simulink model "sampleModel1960"  (R2023a)
settings: Solver=VariableStepAuto  StartTime=0.0  StopTime=10.0  RelTol=1e-3
libraries: hdlsllib x4, simulink x2
settings Model: Creator=user1  LastModifiedBy=user1

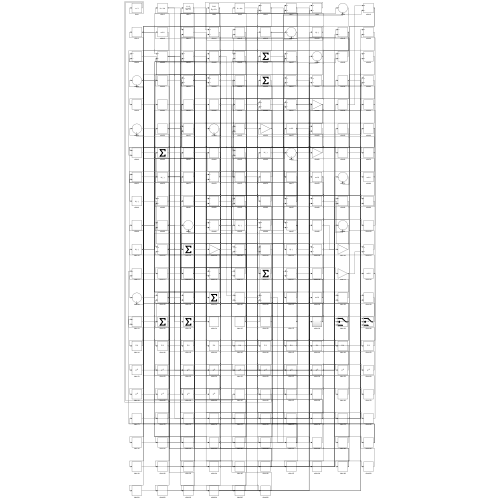
[thumbnail: Simulink's stored preview of the top-level diagram]
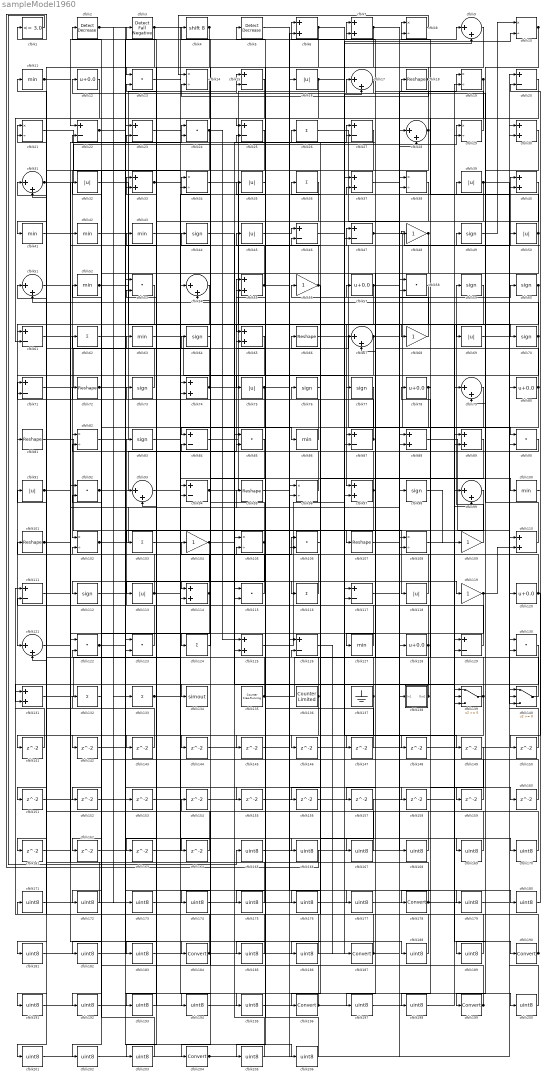
== system sampleModel1960 ==
  cfblk1 : hdlsllib/Logic and Bit Operations/Compare To Constant  relop=<=  const=3.0  OutDataTypeStr=boolean
  cfblk{8,10,14,19,21,29,34,38,82,96,102,105,108} (13 alike) : Product  Inputs=*/  RndMeth=Zero  SaturateOnIntegerOverflow=on
  cfblk{11,41..43,52,63,86,100,127} (9 alike) : MinMax
  cfblk{18,66,72,81,95,101,107} (7 alike) : Reshape
  cfblk{26,36,62,103,116,124,132..133} (8 alike) : Sum  Inputs=+
  cfblk{48,56,68,104,109,119} (6 alike) : Gain
  cfblk{13,24,53,58,85,90,92,106,115,122..123,130} (12 alike) : DotProduct  OutDataTypeStr=Inherit: Inherit via internal rule
  cfblk{6..7,30,33,37,40,55,65,74,88..89,97,110,114,125,131} (16 alike) : Sum
  cfblk{15,20,22..23,25,27,46..47,61,71,84,87,94,111,117,126,129} (17 alike) : Sum  Inputs=+-
  cfblk{44,49,59..60,64,70,73,76..77,83,98,112} (12 alike) : Signum
  cfblk{16,32,35,39,45,50,69,75,91,113,118} (11 alike) : Abs  SaturateOnIntegerOverflow=off
  cfblk{12,57,78,80,120,128} (6 alike) : Bias  Bias=0.0  SaturateOnIntegerOverflow=off
  cfblk{9,17,28,31,51,54,67,79,93,99,121} (11 alike) : Sum  Inputs=|++
  cfblk134 : ToWorkspace  VariableName=simout  SaveFormat=Timeseries  SampleTime=-1
  cfblk135 : hdlsllib/Sources/Counter Free-Running  NumBits=16  tsamp=-1
  cfblk136 : hdlsllib/Sources/Counter Limited  uplimit=7  tsamp=-1
  cfblk137 : Ground
  cfblk138 : Subsystem
      settings: LibrarySourceBlock=|
      | hdlsllib/Ports &
      | Subsystems/Subsystem
  cfblk139 : Switch  SaturateOnIntegerOverflow=off  InputSameDT=off
  cfblk140 : Switch  SaturateOnIntegerOverflow=off  InputSameDT=off
  cfblk{141..164} (24 alike) : Delay  SampleTime=1
  cfblk{165..177,179..183,185..186,188..189,191..195,197..198,200..203,205..206} (35 alike) : DataTypeConversion  OutDataTypeStr=uint8  SaturateOnIntegerOverflow=off  RndMeth=Floor
  cfblk{178,184,187,190,196,199,204} (7 alike) : DataTypeConversion  SaturateOnIntegerOverflow=off  RndMeth=Floor
  cfblk2 : simulink/Logic and Bit Operations/Detect Decrease  vinit=0.0  OutDataTypeStr=boolean
      settings: LibrarySourceBlock=|
      | hdlsllib/Logic and Bit
      | Operations/Detect
      | Decrease
  cfblk3 : hdlsllib/Logic and Bit Operations/Detect Fall Negative  vinit=0  OutDataTypeStr=boolean
  cfblk4 : ArithShift  BitShiftNumber=8
  cfblk5 : simulink/Logic and Bit Operations/Detect Decrease  vinit=0.0  OutDataTypeStr=boolean
      settings: LibrarySourceBlock=|
      | hdlsllib/Logic and Bit
      | Operations/Detect
      | Decrease
  wires:
  cfblk116/1 -> cfblk104/1
  cfblk74/1 -> cfblk17/1, cfblk31/1
  cfblk82/1 -> cfblk15/1
  cfblk98/1 -> cfblk109/1
  cfblk124/1 -> cfblk4/1
  cfblk17/1 -> cfblk15/2
  cfblk123/1 -> cfblk83/1
  cfblk54/1 -> cfblk121/1
  cfblk8/1 -> cfblk14/1
  cfblk47/1 -> cfblk90/1, cfblk19/1
  cfblk68/1 -> cfblk56/1
  cfblk65/1 -> cfblk81/1
  cfblk100/1 -> cfblk48/1
  cfblk66/1 -> cfblk90/2
  cfblk75/1 -> cfblk96/2, cfblk115/2
  cfblk24/1 -> cfblk102/1, cfblk125/1
  cfblk81/1 -> cfblk118/1
  cfblk32/1 -> cfblk97/1
  cfblk34/1 -> cfblk68/1
  cfblk29/1 -> cfblk6/1
  cfblk31/1 -> cfblk29/1, cfblk124/1
  cfblk49/1 -> cfblk10/1
  cfblk136/1 -> cfblk55/2, cfblk191/1
  cfblk87/1 -> cfblk71/1, cfblk46/2
  cfblk30/1 -> cfblk199/1
  cfblk85/1 -> cfblk204/1
  cfblk94/1 -> cfblk10/2, cfblk27/1
  cfblk109/1 -> cfblk59/1
  cfblk92/1 -> cfblk55/1, cfblk133/1
  cfblk61/1 -> cfblk82/1
  cfblk131/1 -> cfblk74/1
  cfblk9/1 -> cfblk25/1
  cfblk78/1 -> cfblk125/2, cfblk148/1
  cfblk76/1 -> cfblk26/1
  cfblk36/1 -> cfblk134/1
  cfblk97/1 -> cfblk23/2, cfblk156/1, cfblk157/1
  cfblk20/1 -> cfblk178/1
  cfblk127/1 -> cfblk93/1
  cfblk120/1 -> cfblk3/1, cfblk150/1
  cfblk22/1 -> cfblk8/2, cfblk153/1, cfblk195/1
  cfblk55/1 -> cfblk45/1, cfblk27/2
  cfblk50/1 -> cfblk8/1, cfblk127/1
  cfblk42/1 -> cfblk129/1
  cfblk28/1 -> cfblk93/2, cfblk18/1
  cfblk64/1 -> cfblk114/1
  cfblk56/1 -> cfblk25/2, cfblk146/1
  cfblk62/1 -> cfblk123/1
  cfblk52/1 -> cfblk120/1, cfblk7/2
  cfblk69/1 -> cfblk110/1
  cfblk86/1 -> cfblk34/1
  cfblk93/1 -> cfblk100/1
  cfblk95/1 -> cfblk47/1
  cfblk140/1 -> cfblk21/1
  cfblk128/1 -> cfblk131/2, cfblk67/2, cfblk101/1
  cfblk96/1 -> cfblk2/1
  cfblk107/1 -> cfblk60/1
  cfblk118/1 -> cfblk76/1
  cfblk114/1 -> cfblk52/1, cfblk182/1
  cfblk103/1 -> cfblk107/1
  cfblk104/1 -> cfblk112/1, cfblk39/1
  cfblk7/1 -> cfblk160/1, cfblk161/1
  cfblk73/1 -> cfblk11/1
  cfblk23/1 -> cfblk34/2
  cfblk88/1 -> cfblk140/3
  cfblk16/1 -> cfblk65/1, cfblk69/1, cfblk9/2
  cfblk26/1 -> cfblk88/1
  cfblk13/1 -> cfblk114/2
  cfblk110/1 -> cfblk12/1
  cfblk119/1 -> cfblk139/2, cfblk110/2
  cfblk84/1 -> cfblk40/1
  cfblk4/1 -> cfblk41/1, cfblk103/1
  cfblk6/1 -> cfblk67/1, cfblk164/1
  cfblk63/1 -> cfblk87/1
  cfblk14/1 -> cfblk113/1
  cfblk122/1 -> cfblk32/1, cfblk158/1
  cfblk3/1 -> cfblk70/1, cfblk151/1
  cfblk108/1 -> cfblk190/1
  cfblk2/1 -> cfblk170/1, cfblk173/1
  cfblk113/1 -> cfblk82/2, cfblk200/1
  cfblk101/1 -> cfblk42/1, cfblk24/2
  cfblk21/1 -> cfblk54/1
  cfblk112/1 -> cfblk119/1
  cfblk121/1 -> cfblk95/1
  cfblk138/1(Out1) -> cfblk122/2, cfblk7/1
  cfblk57/1 -> cfblk159/1, cfblk201/1
  cfblk89/1 -> cfblk196/1
  cfblk44/1 -> cfblk139/3
  cfblk71/1 -> cfblk40/2
  cfblk33/1 -> cfblk97/2, cfblk86/1
  cfblk139/1 -> cfblk66/1, cfblk78/1, cfblk147/1, cfblk185/1
  cfblk67/1 -> cfblk38/2, cfblk77/1
  cfblk111/1 -> cfblk184/1
  cfblk129/1 -> cfblk57/1
  cfblk51/1 -> cfblk129/2
  cfblk125/1 -> cfblk17/2
  cfblk60/1 -> cfblk121/2, cfblk194/1
  cfblk45/1 -> cfblk46/1
  cfblk70/1 -> cfblk75/1, cfblk51/2
  cfblk80/1 -> cfblk84/1, cfblk22/2
  cfblk137/1 -> cfblk51/1, cfblk92/2, cfblk174/1
  cfblk102/1 -> cfblk28/1, cfblk116/1, cfblk162/1
  cfblk72/1 -> cfblk64/1, cfblk106/2, cfblk177/1
  cfblk25/1 -> cfblk61/1
  cfblk39/1 -> cfblk80/1, cfblk54/2
  cfblk10/1 -> cfblk79/2, cfblk189/1
  cfblk41/1 -> cfblk123/2
  cfblk133/1 -> cfblk37/2, cfblk106/1
  cfblk48/1 -> cfblk142/1, cfblk203/1
  cfblk135/1 -> cfblk33/1, cfblk28/2
  cfblk12/1 -> cfblk61/2
  cfblk19/1 -> cfblk94/2, cfblk144/1
  cfblk90/1 -> cfblk84/2
  cfblk18/1 -> cfblk14/2, cfblk13/1
  cfblk91/1 -> cfblk24/1, cfblk49/1
  cfblk115/1 -> cfblk71/2
  cfblk126/1 -> cfblk187/1
  cfblk11/1 -> cfblk22/1, cfblk9/1
  cfblk105/1 -> cfblk44/1, cfblk183/1
  cfblk15/1 -> cfblk141/1
  cfblk141/1 -> cfblk131/1
  cfblk40/1 -> cfblk143/1
  cfblk143/1 -> cfblk21/2
  cfblk144/1 -> cfblk6/2
  cfblk35/1 -> cfblk145/1
  cfblk146/1 -> cfblk79/1
  cfblk147/1 -> cfblk65/2
  cfblk148/1 -> cfblk140/1
  cfblk46/1 -> cfblk149/1
  cfblk150/1 -> cfblk140/2
  cfblk151/1 -> cfblk47/2
  cfblk27/1 -> cfblk152/1
  cfblk152/1 -> cfblk96/1
  cfblk153/1 -> cfblk94/1
  cfblk154/1 -> cfblk139/1
  cfblk43/1 -> cfblk155/1
  cfblk155/1 -> cfblk29/2
  cfblk156/1 -> cfblk38/1
  cfblk158/1 -> cfblk19/2
  cfblk159/1 -> cfblk102/2
  cfblk160/1 -> cfblk105/1
  cfblk77/1 -> cfblk163/1
  cfblk163/1 -> cfblk74/2
  cfblk164/1 -> cfblk31/2
  cfblk1/1 -> cfblk165/1
  cfblk165/1 -> cfblk128/1
  cfblk162/1 -> cfblk166/1
  cfblk166/1 -> cfblk1/1
  cfblk5/1 -> cfblk167/1
  cfblk167/1 -> cfblk35/1
  cfblk37/1 -> cfblk168/1
  cfblk168/1 -> cfblk5/1
  cfblk117/1 -> cfblk169/1
  cfblk169/1 -> cfblk92/1
  cfblk170/1 -> cfblk117/1
  cfblk171/1 -> cfblk117/2
  cfblk130/1 -> cfblk172/1
  cfblk172/1 -> cfblk122/1
  cfblk173/1 -> cfblk130/1
  cfblk174/1 -> cfblk130/2
  cfblk58/1 -> cfblk175/1
  cfblk175/1 -> cfblk73/1
  cfblk106/1 -> cfblk176/1
  cfblk176/1 -> cfblk58/1
  cfblk177/1 -> cfblk58/2
  cfblk178/1 -> cfblk33/2, cfblk91/1
  cfblk145/1 -> cfblk179/1
  cfblk179/1 -> cfblk20/1
  cfblk83/1 -> cfblk180/1
  cfblk180/1 -> cfblk20/2
  cfblk53/1 -> cfblk181/1
  cfblk181/1 -> cfblk138/1(In1)
  cfblk182/1 -> cfblk53/1
  cfblk183/1 -> cfblk53/2
  cfblk184/1 -> cfblk13/2, cfblk87/2
  cfblk185/1 -> cfblk111/1
  cfblk157/1 -> cfblk186/1
  cfblk186/1 -> cfblk111/2
  cfblk187/1 -> cfblk171/1, cfblk105/2, cfblk115/1
  cfblk161/1 -> cfblk188/1
  cfblk188/1 -> cfblk126/1
  cfblk189/1 -> cfblk126/2
  cfblk190/1 -> cfblk36/1, cfblk23/1, cfblk37/1
  cfblk191/1 -> cfblk108/1
  cfblk79/1 -> cfblk192/1
  cfblk192/1 -> cfblk108/2
  cfblk99/1 -> cfblk193/1
  cfblk193/1 -> cfblk63/1
  cfblk194/1 -> cfblk99/1
  cfblk195/1 -> cfblk99/2
  cfblk196/1 -> cfblk72/1, cfblk62/1
  cfblk59/1 -> cfblk197/1
  cfblk197/1 -> cfblk89/1
  cfblk149/1 -> cfblk198/1
  cfblk198/1 -> cfblk89/2
  cfblk199/1 -> cfblk154/1, cfblk43/1
  cfblk200/1 -> cfblk30/1
  cfblk201/1 -> cfblk30/2
  cfblk132/1 -> cfblk202/1
  cfblk202/1 -> cfblk16/1
  cfblk203/1 -> cfblk132/1
  cfblk204/1 -> cfblk50/1, cfblk88/2, cfblk98/1
  cfblk38/1 -> cfblk205/1
  cfblk205/1 -> cfblk85/1
  cfblk142/1 -> cfblk206/1
  cfblk206/1 -> cfblk85/2

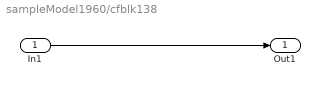
== system sampleModel1960/cfblk138 ==
  In1 : Inport
  Out1 : Outport
  wires:
  In1/1 -> Out1/1
